simulink model "Simulazione_cascata"  (R2023b)
settings: Solver=VariableStepAuto  StartTime=0.0  StopTime=20  RelTol=1e-3
values from neighbouring files (symbols this model uses):
  den_mag_C2 = Gden{1}    [Controllo_un_anello_v2.m]    (also in Controllore_testato.m; controllo_un_anello.m)
  lower = 0    [Controllo_un_anello_v2.m]    (also in Controllore_testato.m; controllo_un_anello.m; controllore_piu_anelli.m)
  Lower_bound_V = -23    [Controllo_un_anello_v2.m]    (also in Controllore_testato.m = 0; controllo_un_anello.m; controllore_piu_anelli.m)
  num_mag_C2 = Gnum{1}    [Controllo_un_anello_v2.m]    (also in Controllore_testato.m; controllo_un_anello.m)
  upper = 12e-3    (= 0.012)    [Controllo_un_anello_v2.m]    (also in Controllore_testato.m; controllo_un_anello.m; controllore_piu_anelli.m)
  Upper_bound_V = 23    [Controllo_un_anello_v2.m]    (also in Controllore_testato.m; controllo_un_anello.m; controllore_piu_anelli.m)
undefined symbols (not defined in the file or in its folder): ki2, kp2, Lc, Rtot
libraries: slpidlib x2, SignalEditorBlockLib x1
settings Model: Creator=lollo  LastModifiedBy=lollo

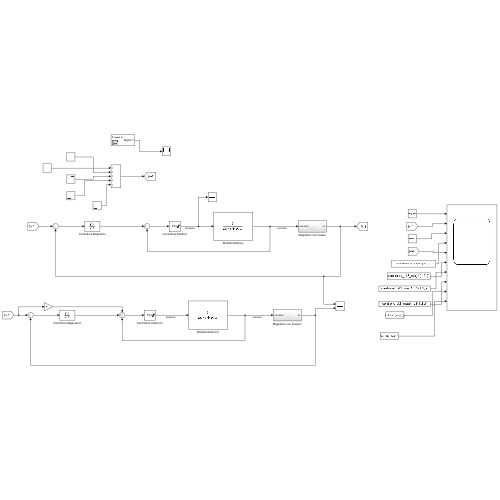
[thumbnail: Simulink's stored preview of the top-level diagram]
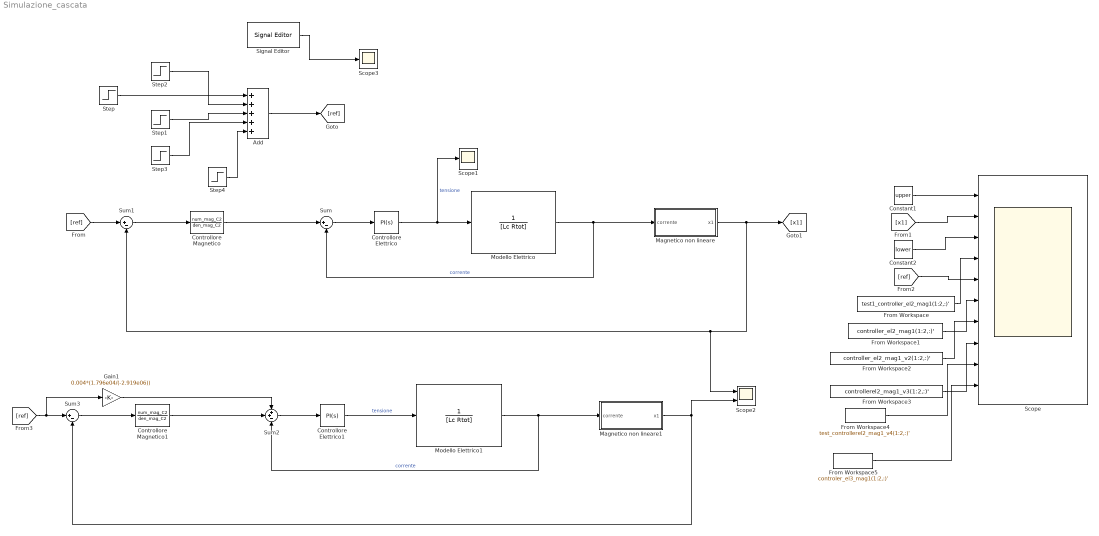
== system Simulazione_cascata ==
  Add : Sum  Inputs=+++++
  Constant1 : Constant  Value=upper
  Constant2 : Constant  Value=lower
  Controllore Elettrico : slpidlib/PID Controller  Controller=PI  Form=Parallel  TimeDomain=Continuous-time  UseExternalTs=off  SampleTime=-1  IntegratorMethod=Forward Euler  FilterMethod=Forward Euler  ControllerParametersSource=internal  P=kp2  I=ki2  UseKiTs=off  D=0  N=100  UseFilter=on  TunerSelectOption=Transfer Function Based (PID Tuner App)  InitialConditionSource=internal  InitialConditionForIntegrator=0  InitialConditionForFilter=0  DifferentiatorICPrevScaledInput=0  ExternalReset=none  TrackingMode=off  Kt=1  LimitOutput=on  SatLimitsSource=internal  UpperSaturationLimit=Upper_bound_V  LowerSaturationLimit=Lower_bound_V  LinearizeAsGain=on  AntiWindupMode=none  Kb=1  LimitIntegrator=off  UpperIntegratorSaturationLimit=inf  LowerIntegratorSaturationLimit=-inf  POutMin=[]  POutMax=[]  IOutMin=[]  IOutMax=[]  DOutMin=[]  DOutMax=[]  NOutMin=[]  NOutMax=[]  SumOutMin=[]  SumOutMax=[]  SaturationOutMin=[]  SaturationOutMax=[]  PParamMin=[]  PParamMax=[]  IParamMin=[]  IParamMax=[]  DParamMin=[]  DParamMax=[]  NParamMin=[]  NParamMax=[]  KbParamMin=[]  KbParamMax=[]  KtParamMin=[]  KtParamMax=[]  KbOutMin=[]  KbOutMax=[]  KtOutMin=[]  KtOutMax=[]  IntegratorOutMin=[]  IntegratorOutMax=[]  FilterOutMin=[]  FilterOutMax=[]  SumI1OutMin=[]  SumI1OutMax=[]  SumI2OutMin=[]  SumI2OutMax=[]  SumI3OutMin=[]  SumI3OutMax=[]  SumI4OutMin=[]  SumI4OutMax=[]  SumDOutMin=[]  SumDOutMax=[]  DifferentiatorOutMin=[]  DifferentiatorOutMax=[]  FilterDiffOutCoefMin=[]  FilterDiffOutCoefMax=[]  ReciprocalOutMin=[]  ReciprocalOutMax=[]  SumDenOutMin=[]  SumDenOutMax=[]  SumNumOutMin=[]  SumNumOutMax=[]  DivideOutMin=[]  DivideOutMax=[]  UdiffTsProdOutMin=[]  UdiffTsProdOutMax=[]  NTsProdOutMin=[]  NTsProdOutMax=[]  UintegralTsProdOutMin=[]  UintegralTsProdOutMax=[]  UngainTsProdOutMin=[]  UngainTsProdOutMax=[]  ClampingZeroOutDataTypeStr=Inherit: Inherit via back propagation  ClampingZeroOutMin=[]  ClampingZeroOutMax=[]  FilterDenConstantOutDataTypeStr=Inherit: Inherit via back propagation  FilterDenConstantOutMin=[]  FilterDenConstantOutMax=[]  PCopyOutDataTypeStr=Inherit: Inherit via back propagation  PCopyOutMin=[]  PCopyOutMax=[]  NCopyOutDataTypeStr=Inherit: Inherit via back propagation  NCopyOutMin=[]  NCopyOutMax=[]  IntegratorContinuousStateAttributes=''  IntegratorStateMustResolveToSignalObject=off  IntegratorRTWStateStorageClass=Auto  FilterContinuousStateAttributes=''  FilterStateMustResolveToSignalObject=off  FilterRTWStateStorageClass=Auto  ParallelPVariant=InternalParameters  IdealPVariant=Disabled  IVariant=InternalParameters  DVariant=Disabled  IntegratorVariant=Continuous  SatVariant=Enabled  AWVariant=Passthrough  PCopyVariant=Disabled  TRVariant=Disabled  FdbkBlocksVariant=Forward  IdealPFdbkVariant=Disabled  SatFdbkVariant=Disabled  DerivativeFilterVariant=Disabled  NVariant=Disabled  NCopyVariant=Disabled_SignalSpec  FilterICVariant=Disabled  IntegratorICVariant=InternalICs  ExternalResetVariant=Disabled  TRSumVariant=Passthrough  SumFdbkVariant=Disabled  SumVariant=Sum_PI  TsampFilterVariant=InternalTs  TsampNgainVariant=Passthrough  TsampIntegralVariant=Disabled_SignalSpec  ExternalSaturationOutDataTypeStr=Inherit: Same as second input
  Controllore Elettrico1 : slpidlib/PID Controller  Controller=PI  Form=Parallel  TimeDomain=Continuous-time  UseExternalTs=off  SampleTime=-1  IntegratorMethod=Forward Euler  FilterMethod=Forward Euler  ControllerParametersSource=internal  P=kp2  I=ki2  UseKiTs=off  D=0  N=100  UseFilter=on  TunerSelectOption=Transfer Function Based (PID Tuner App)  InitialConditionSource=internal  InitialConditionForIntegrator=0  InitialConditionForFilter=0  DifferentiatorICPrevScaledInput=0  ExternalReset=none  TrackingMode=off  Kt=1  LimitOutput=on  SatLimitsSource=internal  UpperSaturationLimit=Upper_bound_V  LowerSaturationLimit=Lower_bound_V  LinearizeAsGain=on  AntiWindupMode=none  Kb=1  LimitIntegrator=off  UpperIntegratorSaturationLimit=inf  LowerIntegratorSaturationLimit=-inf  POutMin=[]  POutMax=[]  IOutMin=[]  IOutMax=[]  DOutMin=[]  DOutMax=[]  NOutMin=[]  NOutMax=[]  SumOutMin=[]  SumOutMax=[]  SaturationOutMin=[]  SaturationOutMax=[]  PParamMin=[]  PParamMax=[]  IParamMin=[]  IParamMax=[]  DParamMin=[]  DParamMax=[]  NParamMin=[]  NParamMax=[]  KbParamMin=[]  KbParamMax=[]  KtParamMin=[]  KtParamMax=[]  KbOutMin=[]  KbOutMax=[]  KtOutMin=[]  KtOutMax=[]  IntegratorOutMin=[]  IntegratorOutMax=[]  FilterOutMin=[]  FilterOutMax=[]  SumI1OutMin=[]  SumI1OutMax=[]  SumI2OutMin=[]  SumI2OutMax=[]  SumI3OutMin=[]  SumI3OutMax=[]  SumI4OutMin=[]  SumI4OutMax=[]  SumDOutMin=[]  SumDOutMax=[]  DifferentiatorOutMin=[]  DifferentiatorOutMax=[]  FilterDiffOutCoefMin=[]  FilterDiffOutCoefMax=[]  ReciprocalOutMin=[]  ReciprocalOutMax=[]  SumDenOutMin=[]  SumDenOutMax=[]  SumNumOutMin=[]  SumNumOutMax=[]  DivideOutMin=[]  DivideOutMax=[]  UdiffTsProdOutMin=[]  UdiffTsProdOutMax=[]  NTsProdOutMin=[]  NTsProdOutMax=[]  UintegralTsProdOutMin=[]  UintegralTsProdOutMax=[]  UngainTsProdOutMin=[]  UngainTsProdOutMax=[]  ClampingZeroOutDataTypeStr=Inherit: Inherit via back propagation  ClampingZeroOutMin=[]  ClampingZeroOutMax=[]  FilterDenConstantOutDataTypeStr=Inherit: Inherit via back propagation  FilterDenConstantOutMin=[]  FilterDenConstantOutMax=[]  PCopyOutDataTypeStr=Inherit: Inherit via back propagation  PCopyOutMin=[]  PCopyOutMax=[]  NCopyOutDataTypeStr=Inherit: Inherit via back propagation  NCopyOutMin=[]  NCopyOutMax=[]  IntegratorContinuousStateAttributes=''  IntegratorStateMustResolveToSignalObject=off  IntegratorRTWStateStorageClass=Auto  FilterContinuousStateAttributes=''  FilterStateMustResolveToSignalObject=off  FilterRTWStateStorageClass=Auto  ParallelPVariant=InternalParameters  IdealPVariant=Disabled  IVariant=InternalParameters  DVariant=Disabled  IntegratorVariant=Continuous  SatVariant=Enabled  AWVariant=Passthrough  PCopyVariant=Disabled  TRVariant=Disabled  FdbkBlocksVariant=Forward  IdealPFdbkVariant=Disabled  SatFdbkVariant=Disabled  DerivativeFilterVariant=Disabled  NVariant=Disabled  NCopyVariant=Disabled_SignalSpec  FilterICVariant=Disabled  IntegratorICVariant=InternalICs  ExternalResetVariant=Disabled  TRSumVariant=Passthrough  SumFdbkVariant=Disabled  SumVariant=Sum_PI  TsampFilterVariant=InternalTs  TsampNgainVariant=Passthrough  TsampIntegralVariant=Disabled_SignalSpec  ExternalSaturationOutDataTypeStr=Inherit: Same as second input
  Controllore Magnetico : TransferFcn  Numerator=num_mag_C2  Denominator=den_mag_C2
  Controllore Magnetico1 : TransferFcn  Numerator=num_mag_C2  Denominator=den_mag_C2
  From Workspace : FromWorkspace  VariableName=test1_controller_el2_mag1(1:2,:)'
  From Workspace1 : FromWorkspace  VariableName=controller_el2_mag1(1:2,:)'
  From Workspace2 : FromWorkspace  VariableName=controller_el2_mag1_v2(1:2,:)'
  From Workspace3 : FromWorkspace  VariableName=controllerel2_mag1_v3(1:2,:)'
  From Workspace4 : FromWorkspace  VariableName=test_controllerel2_mag1_v4(1:2,:)'
  From Workspace5 : FromWorkspace  VariableName=controler_el3_mag1(1:2,:)'
  Gain1 : Gain  Gain=0.004*(1.796e04/(-2.919e06))
  Magnetico non lineare : Subsystem
  Magnetico non lineare1 : Subsystem
  Modello Elettrico : TransferFcn  Denominator=[Lc Rtot]
  Modello Elettrico1 : TransferFcn  Denominator=[Lc Rtot]
  Scope : Scope  NumInputPorts=10
  Scope1 : Scope
  Scope2 : Scope  NumInputPorts=2
  Scope3 : Scope
  Signal Editor : SignalEditorBlockLib/Signal Editor  FileName=untitled.mat  ActiveScenario=Scenario  ActiveSignal=Signal 1  IsBus=off  OutputBusObjectStr=Bus: BusObject  SampleTime=0  Interpolate=off  ZeroCross=off  OutputAfterFinalValue=Setting to zero  Unit=inherit  PreserveSignalName=on  ApplySigPropsToAllScenarios=on  ApplySigPropsToAllSignals=off
  Step : Step  Time=0  After=0.001  SampleTime=0
  Step1 : Step  Time=5  After=0.001  SampleTime=0
  Step2 : Step  Time=7  After=0.001  SampleTime=0
  Step3 : Step  Time=9  After=0.001  SampleTime=0
  Step4 : Step  Time=11  After=0.001  SampleTime=0
  Sum : Sum  Inputs=|+-
  Sum1 : Sum  Inputs=|+-
  Sum2 : Sum  Inputs=++-
  Sum3 : Sum  Inputs=|+-
  wires:
  Sum/1 -> Controllore Elettrico/1
  Controllore Magnetico/1 -> Sum/1
  Controllore Elettrico/1 -> Scope1/1, Modello Elettrico/1  "tensione"
  Modello Elettrico/1 -> Sum/2, Magnetico non lineare/1(corrente)  "corrente"
  Sum1/1 -> Controllore Magnetico/1
  [ref] -> Sum1/1
  Constant1/1 -> Scope/1
  [x1] -> Scope/2
  Constant2/1 -> Scope/3
  [ref] -> Scope/5
  Step/1 -> Add/1
  Signal Editor/1 -> Scope3/1
  Step1/1 -> Add/3
  Step2/1 -> Add/2
  Step3/1 -> Add/4
  Step4/1 -> Add/5
  From Workspace/1 -> Scope/4
  From Workspace1/1 -> Scope/6
  From Workspace2/1 -> Scope/7
  From Workspace3/1 -> Scope/8
  From Workspace4/1 -> Scope/9
  From Workspace5/1 -> Scope/10
  Magnetico non lineare/1(x1) -> Scope2/1, Sum1/2, [x1]
  Controllore Magnetico1/1 -> Sum2/2
  Gain1/1 -> Sum2/1
  Controllore Elettrico1/1 -> Modello Elettrico1/1  "tensione"
  Magnetico non lineare1/1(x1) -> Scope2/2, Sum3/2
  [ref] -> Gain1/1, Sum3/1
  Sum3/1 -> Controllore Magnetico1/1
  Modello Elettrico1/1 -> Sum2/3, Magnetico non lineare1/1(corrente)  "corrente"
  Sum2/1 -> Controllore Elettrico1/1
  Add/1 -> [ref]

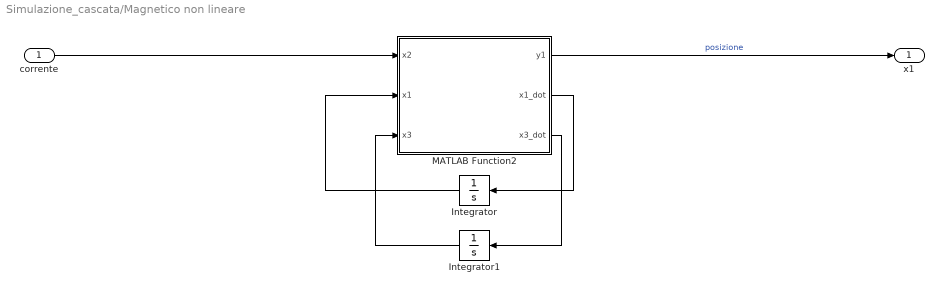
== system Simulazione_cascata/Magnetico non lineare ==
  corrente : Inport
  Integrator : Integrator
  Integrator1 : Integrator
  MATLAB Function2 : MATLAB Function  TreatAsAtomicUnit=on
  x1 : Outport
  wires:
  corrente/1 -> MATLAB Function2/1(x2)
  MATLAB Function2/1(y1) -> x1/1  "posizione"
  MATLAB Function2/2(x1_dot) -> Integrator/1
  Integrator/1 -> MATLAB Function2/2(x1)
  MATLAB Function2/3(x3_dot) -> Integrator1/1
  Integrator1/1 -> MATLAB Function2/3(x3)

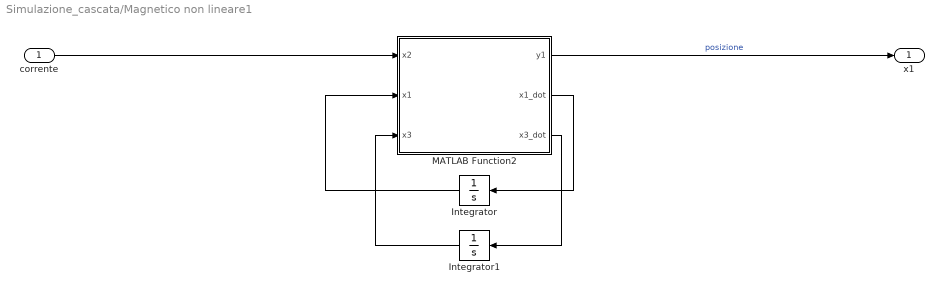
== system Simulazione_cascata/Magnetico non lineare1 ==
  corrente : Inport
  Integrator : Integrator
  Integrator1 : Integrator
  MATLAB Function2 : MATLAB Function  TreatAsAtomicUnit=on
  x1 : Outport
  wires:
  corrente/1 -> MATLAB Function2/1(x2)
  MATLAB Function2/1(y1) -> x1/1  "posizione"
  MATLAB Function2/2(x1_dot) -> Integrator/1
  Integrator/1 -> MATLAB Function2/2(x1)
  MATLAB Function2/3(x3_dot) -> Integrator1/1
  Integrator1/1 -> MATLAB Function2/3(x3)

== matlab function Simulazione_cascata/Magnetico non lineare1/MATLAB Function2 ==
  data: y1 output; x2 input; x1_dot output; x1 input; x3 input; x3_dot output
function [y1,x1_dot, x3_dot] = fcn(x2, x1, x3)
    m = 0.0657;
    g = 9.81;
    k_mag = 2.4405e-05;
    Rtot = 9.7585;
    Lc = 0.3708;
    y0 = 0.012;
    
    x1_dot = x3;
    if x1 < y0
        x3_dot = (k_mag/m)*(x2/(y0-x1))^2 - g;
    else
        x1 = 0.012;
        x3_dot = 0;
        x3 = 0;
    end

    
    % condizioni
    if x1 <=0 && x3_dot < 0
        x1 = 0;
        x3 = 0;
        x3_dot = 0;
    end
y1 = x1;

== matlab function Simulazione_cascata/Magnetico non lineare/MATLAB Function2 ==
  data: y1 output; x2 input; x1_dot output; x1 input; x3 input; x3_dot output
function [y1,x1_dot, x3_dot] = fcn(x2, x1, x3)
    m = 0.0657;
    g = 9.81;
    k_mag = 2.4405e-05;
    Rtot = 9.7585;
    Lc = 0.3708;
    y0 = 0.012;
    
    x1_dot = x3;
    if x1 < y0
        x3_dot = (k_mag/m)*(x2/(y0-x1))^2 - g;
    else
        x1 = 0.012;
        x3_dot = 0;
        x3 = 0;
    end

    
    % condizioni
    if x1 <=0 && x3_dot < 0
        x1 = 0;
        x3 = 0;
        x3_dot = 0;
    end
y1 = x1;
